simulink model "VINS"  (R2018a)
settings: Solver=FixedStepDiscrete  StartTime=0.0  StopTime=inf  FixedStep=1/Fs  RelTol=1e-3  EnableMultiTasking=on
PreLoadFcn:
  | modelDef = getModelDef(calibrateSFMA);
  | 
  | %imuPar = getImuPar('lmvpUncalibrated');
  | 
  | timeMatchThreshold = 1000;
undefined symbols (not defined in the file or in its folder): beep, dejitter_on, Fs, homogeneous3x4Transform_k_kmin1, imuLocationMm, imuPar, numStates, simData, tstamp_k_us, tstamp_kmin1_us
libraries: simulink x69, dspmtrx3 x35, dspindex x9, vrlib x7, dspstat3 x7, dspinverses x6, dspsigops x5, dspmathops x2, rtwdemowidgets x1, dspfactors x1, simulink_extras x1
(part 6 of 6)

== matlab function VINS/measUpdate/absolutePoseUpdate/updateCovariance/modifiedCholesky ==
  data: G input; L output; D output; E output
%
%  [L,D,E,pneg]=mchol(G)
%
%  Given a symmetric matrix G, find a matrix E of "small" norm and c
%  L, and D such that  G+E is Positive Definite, and 
%
%      G+E = L*D*L'
%
%  Also, calculate a direction pneg, such that if G is not PD, then
%
%      pneg'*G*pneg < 0
%
%  Note that if G is PD, then the routine will return pneg=[]. 
%
%  Reference: Gill, Murray, and Wright, "Practical Optimization", p111.
%  Author: Brian Borchers (borchers@nmt.edu)
%
function [L,D,E]=mchol(G)
%
%  n gives the size of the matrix.
%
n=size(G,1);
%
%  gamma, zi, nu, and beta2 are quantities used by the algorithm.  
%
gamma=max(diag(G));
zi=max(max(G-diag(diag(G))));
nu=max([1,sqrt(n^2-1)]);
beta2=max([gamma, zi/nu, 1.0E-15]);
%
%  Initialize diag(C) to diag(G).
%
C=diag(diag(G));
%
%  Loop through, calculating column j of L for j=1:n
%

L=zeros(n, 'like', G);
D=zeros(n, 'like', G);
E=zeros(n, 'like', G);

for j=1:n
    %
    %  Calculate the jth row of L.  
    %
    if (j > 1)
        L(j,1:j-1)=C(j,1:j-1)./diag(D(1:j-1,1:j-1))';
    end
    %
    %  Update the jth column of C.
    %
    if (j >= 2)
        if (j < n)
            C(j+1:n,j)=G(j+1:n,j)-(L(j,1:j-1)*C(j+1:n,1:j-1)')';
        end
    else
        C(j+1:n,j)=G(j+1:n,j);
    end
    %
    % Update theta. 
    %
    if (j == n)
        theta_j=cast(0, 'like', G);
    else
        theta_j=max(abs(C(j+1:n,j)));
    end
    %
    %  Update D
    %
    D(j,j)=max([eps,abs(C(j,j)),theta_j^2/beta2]');
    %
    % Update E.
    %
    E(j,j)=D(j,j)-C(j,j);

    
    %
    %  Update C again...
    % 
    %%%%%%%% M.Zibulevsky: begin of changes, old version is commented %%%%%%%%%%%%%
    
    %for i=j+1:n,
    %    C(i,i)=C(i,i)-C(i,j)^2/D(j,j);
    %end;
    
    ind=[j*(n+1)+1 : n+1 : n*n]';
    C(ind)=C(ind)-(1/D(j,j))*C(j+1:n,j).^2;


end

%
% Put 1's on the diagonal of L
%
%for j=1:n,
%    L(j,j)=1;
%end;

ind=[1 : n+1 : n*n]';
L(ind)=cast(1, 'like', G);


return

== matlab function VINS/measUpdate/relocalize/Subsystem/setYaw/MATLAB Function3 ==
  data: Cbn input; eul output size=[3,1]
function eul = dcm2euler(Cbn)

%DCM is Cbn (transforms vectors from b to n)
%eul defined as zyx sequence (yaw,pitch,roll),  but listed in
%roll,pitch,yaw order


pitch=asin(-Cbn(3,1));  %pitch is assumed to be [-pi pi]. singular at pi. use ad-hoc methods to remedy this deficiency
roll=atan2(Cbn(3,2), Cbn(3,3));
heading = atan2(Cbn(2,1), Cbn(1,1));
eul=[roll;pitch;heading];

== matlab function VINS/measUpdate/relocalize/Subsystem/setYaw/euler2dcm ==
  data: eul_vect input; DCMnb output
function DCMnb = eulr2dcm(eul_vect)
%EULR2DCM       Euler angle vector to direction cosine
%               matrix conversion.
%       
%	DCMnb = eulr2dcm(eul_vect)
%
%   INPUTS
%       eul_vect(1) = roll angle in radians 
%
%       eul_vect(2) = pitch angle in radians 
%
%       eul_vect(3) = yaw angle in radians 
%
%   OUTPUTS
%       DCMnb = 3x3 direction cosine matrix providing the
%             transformation from the navigation frame
%             to the body frame
%

%   REFERENCE:  Titterton, D. and J. Weston, STRAPDOWN
%               INERTIAL NAVIGATION TECHNOLOGY, Peter
%               Peregrinus Ltd. on behalf of the Institution
%               of Electrical Engineers, London, 1997.
%
%	M. & S. Braasch 12-97
%	Copyright (c) 1997 by GPSoft
%	All Rights Reserved.
%

  if nargin<1,error('insufficient number of input arguments'),end

  phi = eul_vect(1); theta = eul_vect(2); psi = eul_vect(3);

  cpsi = cos(psi); spsi = sin(psi);
  cthe = cos(theta); sthe = sin(theta);
  cphi = cos(phi); sphi = sin(phi);

  C1 = [cpsi  spsi 0; ...
        -spsi cpsi 0; ...
         0     0   1];
  C2 = [cthe  0  -sthe; ...
          0   1     0 ; ...
        sthe  0   cthe];
  C3 = [1   0    0;   ...
        0  cphi sphi; ...
        0 -sphi cphi];  

  DCMnb = C3 * C2 * C1;

== matlab function VINS/measUpdate/relocalize/Subsystem/MATLAB Function3 ==
  data: Cbn input; eul output size=[3,1]
function eul = dcm2euler(Cbn)

%DCM is Cbn (transforms vectors from b to n)
%eul defined as zyx sequence (yaw,pitch,roll),  but listed in
%roll,pitch,yaw order


pitch=asin(-Cbn(3,1));  %pitch is assumed to be [-pi pi]. singular at pi. use ad-hoc methods to remedy this deficiency
roll=atan2(Cbn(3,2), Cbn(3,3));
heading = atan2(Cbn(2,1), Cbn(1,1));
eul=[roll;pitch;heading];

== matlab function VINS/measUpdate/relocalize/Subsystem/MATLAB Function1 ==
  data: Cbn input; eul output size=[3,1]
function eul = dcm2euler(Cbn)

%DCM is Cbn (transforms vectors from b to n)
%eul defined as zyx sequence (yaw,pitch,roll),  but listed in
%roll,pitch,yaw order


pitch=asin(-Cbn(3,1));  %pitch is assumed to be [-pi pi]. singular at pi. use ad-hoc methods to remedy this deficiency
roll=atan2(Cbn(3,2), Cbn(3,3));
heading = atan2(Cbn(2,1), Cbn(1,1));
eul=[roll;pitch;heading];

== matlab function VINS/measUpdate/commanded reloc/setYaw1/euler2dcm ==
  data: eul_vect input; DCMnb output
function DCMnb = eulr2dcm(eul_vect)
%EULR2DCM       Euler angle vector to direction cosine
%               matrix conversion.
%       
%	DCMnb = eulr2dcm(eul_vect)
%
%   INPUTS
%       eul_vect(1) = roll angle in radians 
%
%       eul_vect(2) = pitch angle in radians 
%
%       eul_vect(3) = yaw angle in radians 
%
%   OUTPUTS
%       DCMnb = 3x3 direction cosine matrix providing the
%             transformation from the navigation frame
%             to the body frame
%

%   REFERENCE:  Titterton, D. and J. Weston, STRAPDOWN
%               INERTIAL NAVIGATION TECHNOLOGY, Peter
%               Peregrinus Ltd. on behalf of the Institution
%               of Electrical Engineers, London, 1997.
%
%	M. & S. Braasch 12-97
%	Copyright (c) 1997 by GPSoft
%	All Rights Reserved.
%

  if nargin<1,error('insufficient number of input arguments'),end

  phi = eul_vect(1); theta = eul_vect(2); psi = eul_vect(3);

  cpsi = cos(psi); spsi = sin(psi);
  cthe = cos(theta); sthe = sin(theta);
  cphi = cos(phi); sphi = sin(phi);

  C1 = [cpsi  spsi 0; ...
        -spsi cpsi 0; ...
         0     0   1];
  C2 = [cthe  0  -sthe; ...
          0   1     0 ; ...
        sthe  0   cthe];
  C3 = [1   0    0;   ...
        0  cphi sphi; ...
        0 -sphi cphi];  

  DCMnb = C3 * C2 * C1;
